simulink library "DYN_TRA"  (Simulink 10.1)
settings: Solver=VariableStepAuto  StartTime=0.0  StopTime=10.0  RelTol=1e-3
undefined symbols (not defined in the file): DYN_TRA_par
settings Model: LogicAnalyzerSignalOrdering=59e064ba-8658-4792-b66c-487750073223  Creator=WilTravis  LastModifiedBy=m_mam

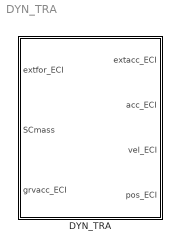
== system DYN_TRA ==
  DYN_TRA : Subsystem

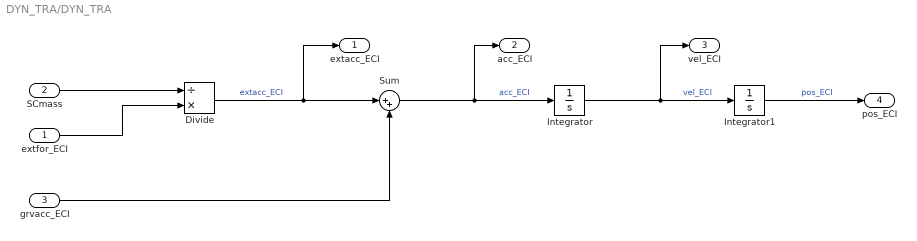
== system DYN_TRA/DYN_TRA ==
  extfor_ECI : Inport
  SCmass : Inport  Port=2
  grvacc_ECI : Inport  Port=3
  Divide : Product  Inputs=/*
  Integrator : Integrator  InitialCondition=DYN_TRA_par.vel_ECI_ini
  Integrator1 : Integrator  InitialCondition=DYN_TRA_par.pos_ECI_ini
  Sum : Sum  Inputs=|++
  extacc_ECI : Outport  VectorParamsAs1DForOutWhenUnconnected=off
  "acc_ECI " : Outport  Port=2  VectorParamsAs1DForOutWhenUnconnected=off
  vel_ECI : Outport  Port=3  VectorParamsAs1DForOutWhenUnconnected=off
  pos_ECI : Outport  Port=4  VectorParamsAs1DForOutWhenUnconnected=off
  wires:
  SCmass/1 -> Divide/1
  Integrator/1 -> Integrator1/1, vel_ECI/1  "vel_ECI"
  Integrator1/1 -> pos_ECI/1  "pos_ECI"
  extfor_ECI/1 -> Divide/2
  Sum/1 -> Integrator/1, "acc_ECI "/1  "acc_ECI"
  grvacc_ECI/1 -> Sum/2
  Divide/1 -> Sum/1, extacc_ECI/1  "extacc_ECI"
